simulink model "target"  (R2018b)
settings: Solver=ode4  StartTime=0.0  StopTime=400  FixedStep=0.03  RelTol=1e-3
values from neighbouring files (symbols this model uses):
  g = 9.8    [init.m]
  init_t = [50000 5000 0 100 deg2rad(30) deg2rad(180)]    [init.m]
libraries: simulink_extras x2
settings Model: Creator=niao4  LastModifiedBy=root
settings RTWCC: TargetLang=C++
settings GRTTargetCC: TargetLangStandard=C++03 (ISO)  MatFileLogging=off  MultiInstanceERTCode=on  CodeInterfacePackaging=C++ class

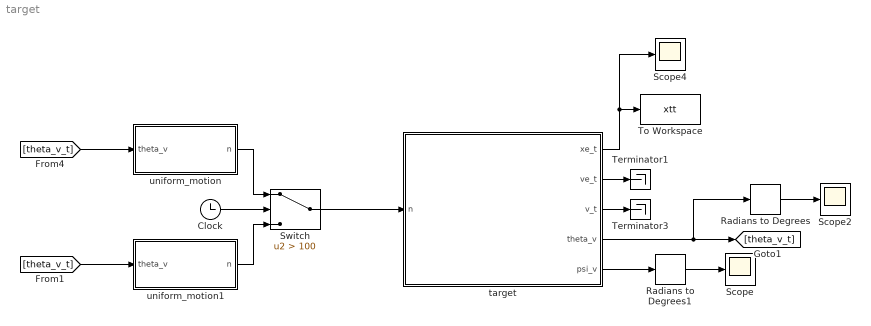
== system target ==
  Clock : Clock
  Radians to Degrees : simulink_extras/Transformations/Radians to Degrees
  Radians to Degrees1 : simulink_extras/Transformations/Radians to Degrees
  Scope : Scope
  Scope2 : Scope
  Scope4 : Scope
  Switch : Switch  Criteria=u2 > Threshold  Threshold=100
  Terminator1 : Terminator
  Terminator3 : Terminator
  To Workspace : ToWorkspace  VariableName=xtt  SampleTime=-1
  target : Subsystem
  uniform_motion : MATLAB Function  TreatAsAtomicUnit=on
  uniform_motion1 : MATLAB Function  TreatAsAtomicUnit=on
  wires:
  target/4(theta_v) -> Radians to Degrees/1, [theta_v_t]
  target/3(v_t) -> Terminator3/1
  target/1(xe_t) -> Scope4/1, To Workspace/1
  target/2(ve_t) -> Terminator1/1
  target/5(psi_v) -> Radians to Degrees1/1
  [theta_v_t] -> uniform_motion/1(theta_v)
  Radians to Degrees/1 -> Scope2/1
  Radians to Degrees1/1 -> Scope/1
  Clock/1 -> Switch/2
  uniform_motion/1(n) -> Switch/1
  uniform_motion1/1(n) -> Switch/3
  [theta_v_t] -> uniform_motion1/1(theta_v)
  Switch/1 -> target/1(n)

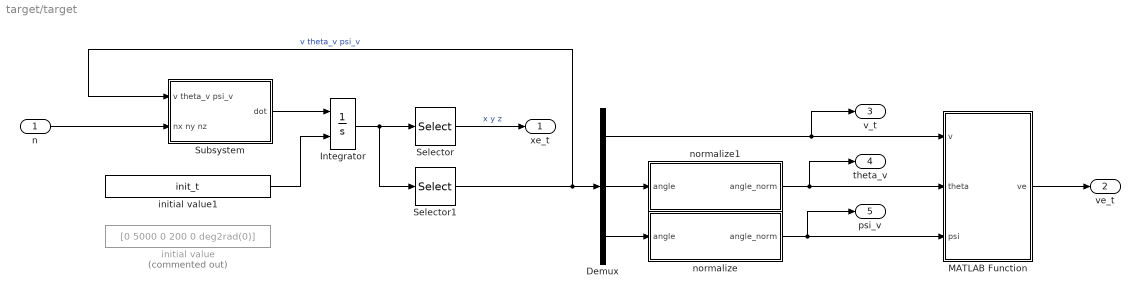
== system target/target ==
  n : Inport
  Demux : Demux  Outputs=3
  Integrator : Integrator  InitialConditionSource=external
  MATLAB Function : MATLAB Function  TreatAsAtomicUnit=on
  Selector : Selector  InputPortWidth=6  IndexOptions=Index vector (dialog)  Indices=[1 2 3]  OutputSizes=1
  Selector1 : Selector  InputPortWidth=6  IndexOptions=Index vector (dialog)  Indices=[4 5 6]  OutputSizes=1
  Subsystem : Subsystem
  initial value : Constant  Commented=on  Value=[0 5000 0 200 0 deg2rad(0)]
  initial value1 : Constant  Value=init_t
  normalize : MATLAB Function  TreatAsAtomicUnit=on
  normalize1 : MATLAB Function  TreatAsAtomicUnit=on
  xe_t : Outport
  ve_t : Outport  Port=2
  v_t : Outport  Port=3
  theta_v : Outport  Port=4
  psi_v : Outport  Port=5
  wires:
  Selector/1 -> xe_t/1  "x y z"
  n/1 -> Subsystem/2(nx ny nz)
  Subsystem/1(dot) -> Integrator/1
  Integrator/1 -> Selector1/1, Selector/1
  Selector1/1 -> Subsystem/1(v theta_v psi_v), Demux/1  "v theta_v psi_v"
  MATLAB Function/1(ve) -> ve_t/1
  Demux/1 -> v_t/1, MATLAB Function/1(v)
  initial value1/1 -> Integrator/2
  Demux/3 -> normalize/1(angle)
  normalize/1(angle_norm) -> psi_v/1, MATLAB Function/3(psi)
  Demux/2 -> normalize1/1(angle)
  normalize1/1(angle_norm) -> theta_v/1, MATLAB Function/2(theta)

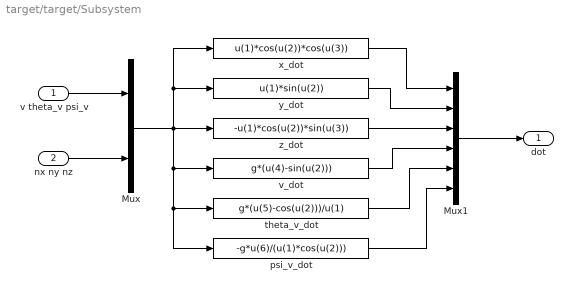
== system target/target/Subsystem ==
  v theta_v psi_v : Inport
  nx ny nz : Inport  Port=2
  Mux : Mux  Inputs=2
  Mux1 : Mux  Inputs=6
  psi_v_dot : Fcn  Expr=-g*u(6)/(u(1)*cos(u(2)))
  theta_v_dot : Fcn  Expr=g*(u(5)-cos(u(2)))/u(1)
  v_dot : Fcn  Expr=g*(u(4)-sin(u(2)))
  x_dot : Fcn  Expr=u(1)*cos(u(2))*cos(u(3))
  y_dot : Fcn  Expr=u(1)*sin(u(2))
  z_dot : Fcn  Expr=-u(1)*cos(u(2))*sin(u(3))
  dot : Outport
  wires:
  theta_v_dot/1 -> Mux1/5
  psi_v_dot/1 -> Mux1/6
  Mux1/1 -> dot/1
  y_dot/1 -> Mux1/2
  Mux/1 -> psi_v_dot/1, theta_v_dot/1, v_dot/1, y_dot/1, x_dot/1, z_dot/1
  x_dot/1 -> Mux1/1
  v_dot/1 -> Mux1/4
  z_dot/1 -> Mux1/3
  nx ny nz/1 -> Mux/2
  v theta_v psi_v/1 -> Mux/1

== matlab function target/normalize1 ==
  data: angle input; angle_norm output
function angle_norm = normalize(angle)
    angle = rad2deg(angle);
    if angle > 180
        angle_norm = angle - floor((angle-(-180))/360)*360;
    elseif angle <= -180
        angle_norm = angle + floor((180-angle)/360)*360;
    else
        angle_norm = angle;
    end
    angle_norm = deg2rad(angle_norm);
end

== matlab function target/normalize ==
  data: angle input; angle_norm output
function angle_norm = normalize(angle)
    angle = rad2deg(angle);
    if angle > 180
        angle_norm = angle - floor((angle-(-180))/360)*360;
    elseif angle <= -180
        angle_norm = angle + floor((180-angle)/360)*360;
    else
        angle_norm = angle;
    end
    angle_norm = deg2rad(angle_norm);
end

== matlab function target/uniform_motion1 ==
  data: theta_v input; n output
function n = uniform(theta_v)
    n = [sin(theta_v) cos(theta_v) 0];
end

== matlab function target/MATLAB Function ==
  data: v input; ve output; theta input; psi input
function ve = v2ve(v, theta, psi)
vx = v * cos(theta) * cos(psi);      
vy = v * sin(theta);      
vz = -v * cos(theta) * sin(psi);
ve = [vx vy vz];
end

== matlab function target/uniform_motion ==
  data: theta_v input; n output
function n = uniform(theta_v)
    n = [sin(theta_v) 1+cos(theta_v) 0];
end
